simulink model "TASK8_1"  (R2019a)
settings: Solver=VariableStepAuto  StartTime=0.0  StopTime=10.0  RelTol=1e-3
values from neighbouring files (symbols this model uses):
  A = [0,mf*g*h/Jconst,0,-(mf*g)/Jconst;1,0,0,0;0,-g,0,0;0,0,1,0]    [Dharmesh_DCS_LAB_Script.m]
  B = [1/Jconst;0;0;0]    [Dharmesh_DCS_LAB_Script.m]
  C = eye(4)    [Dharmesh_DCS_LAB_Script.m]
  D = [0;0;0;0]    [Dharmesh_DCS_LAB_Script.m]
  h1 = ((Kalpha_o)*(Qt_o))    [Dharmesh_DCS_LAB_Script.m]
  K = q * (alpha(5)*eye(4) + alpha(4)*A + alpha(3)*A^2 + alpha(2)*A^3 + A^4)    [Dharmesh_DCS_LAB_Script.m]
  P = 1/(Ct*inv((B*K)-A)*B)    [Dharmesh_DCS_LAB_Script.m]
settings Model: Creator=Admin  LastModifiedBy=Admin

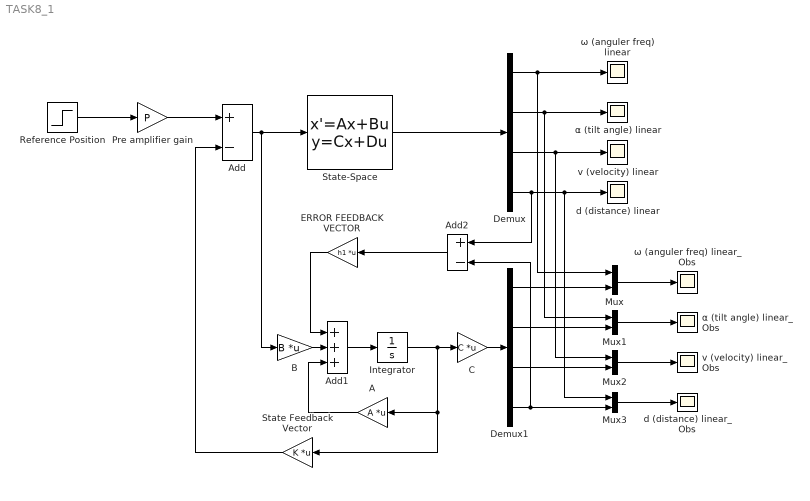
== system TASK8_1 ==
  A : Gain  Gain=A  Multiplication=Matrix(K*u) (u vector)
  Add : Sum  Inputs=+-
  Add1 : Sum  Inputs=+++
  Add2 : Sum  Inputs=+-
  B : Gain  Gain=B  Multiplication=Matrix(K*u) (u vector)
  C : Gain  Gain=C  Multiplication=Matrix(K*u) (u vector)
  Demux : Demux
  Demux1 : Demux
  ERROR FEEDBACK VECTOR : Gain  Gain=h1  Multiplication=Matrix(K*u) (u vector)
  Integrator : Integrator  InitialCondition=[0;0;0;2]
  Mux{,1..3} (4 alike) : Mux  Inputs=2
  Pre amplifier gain : Gain  Gain=P
  Reference Position : Step  Time=0  SampleTime=0
  State Feedback Vector : Gain  Gain=K  Multiplication=Matrix(K*u) (u vector)
  State-Space : StateSpace  A=A  B=B  C=C  D=D  InitialCondition=0
  d (distance) linear : Scope
  d (distance) linear_Obs : Scope
  v (velocity) linear : Scope
  v (velocity) linear_Obs : Scope
  α (tilt angle) linear : Scope
  α (tilt angle) linear_Obs : Scope
  ω (anguler freq) linear : Scope
  ω (anguler freq) linear_Obs : Scope
  wires:
  Demux/2 -> Mux1/1, α (tilt angle) linear/1
  Demux/1 -> Mux/1, ω (anguler freq) linear/1
  State-Space/1 -> Demux/1
  Demux/4 -> Add2/1, Mux3/1, d (distance) linear/1
  Demux/3 -> Mux2/1, v (velocity) linear/1
  Add/1 -> State-Space/1, B/1
  Pre amplifier gain/1 -> Add/1
  Reference Position/1 -> Pre amplifier gain/1
  Add1/1 -> Integrator/1
  A/1 -> Add1/3
  B/1 -> Add1/2
  Integrator/1 -> A/1, State Feedback Vector/1, C/1
  Add2/1 -> ERROR FEEDBACK VECTOR/1
  Demux1/1 -> Mux/2
  Demux1/2 -> Mux1/2
  Demux1/3 -> Mux2/2
  Mux/1 -> ω (anguler freq) linear_Obs/1
  Mux1/1 -> α (tilt angle) linear_Obs/1
  Mux3/1 -> d (distance) linear_Obs/1
  Mux2/1 -> v (velocity) linear_Obs/1
  State Feedback Vector/1 -> Add/2
  ERROR FEEDBACK VECTOR/1 -> Add1/1
  C/1 -> Demux1/1
  Demux1/4 -> Mux3/2, Add2/2
